simulink model "problemm_8"  (R2020b)
settings: Solver=VariableStepAuto  StartTime=0.0  StopTime=10.0  RelTol=1e-3
settings Model: Creator=hp  LastModifiedBy=hp

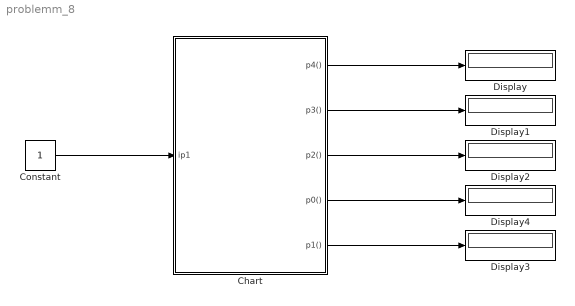
== system problemm_8 ==
  Chart : Stateflow chart  TreatAsAtomicUnit=on
  Constant : Constant
  Display{,1..4} (5 alike) : Display
  wires:
  Constant/1 -> Chart/1(ip1)
  Chart/5(p1()) -> Display3/1
  Chart/4(p0()) -> Display4/1
  Chart/3(p2()) -> Display2/1
  Chart/2(p3()) -> Display1/1
  Chart/1(p4()) -> Display/1

== stateflow chart problemm_8/Chart ==
  state Counter [parallel]
    settings: executionOrder=1
    state init
      en:
      i=0;
    state Count
      en:
      i=ip1
    (default) -> init
    init -> Count
    Count -> Count
  state Action [parallel]
    settings: executionOrder=2
    state Ground
      en:p0;
      during:p0;
    state Fourth
      en:p4;
      during:p4;
    state First
      en:p1;
      during:p1;
    state Third_
      en:p3;
      during:p3
    state Second
      en:p2;
      during:p2;
    (default) -> Ground
    Fourth -> Ground : [ip1==0]
    Ground -> First : [ip1==1]
    Third_ -> Fourth : [ip1==4]
    First -> Second : [ip1==2]
    Second -> Third_ : [ip1==3]
  (default) -> Counter
  data: ip1 input; i constant double
  events: p4 output FUNCTION_CALL_EVENT; p3 output FUNCTION_CALL_EVENT; p2 output FUNCTION_CALL_EVENT; p0 output FUNCTION_CALL_EVENT; p1 output FUNCTION_CALL_EVENT
